simulink model "uniciclo_clot"  (R2020a)
settings: Solver=VariableStepAuto  StartTime=0.0  StopTime=Inf  MaxStep=0.01  RelTol=1e-3
InitFcn:
  | init_uniciclo
StopFcn:
  | stop_uniciclo
values from neighbouring files (symbols this model uses):
  centro = [points(1); points(2)]    [init_uniciclo.m]
  dir_retta = [cos(pi/4); sin(pi/4)]    [init_uniciclo.m]
  K1 = [40; 40]    [init_uniciclo.m]
  K2 = [50; 50]    [init_uniciclo.m]
  Lsofar = [Lsofar; sum(Lenghts)]    [init_uniciclo.m]
  Ltot = sum(Lenghts)    [init_uniciclo.m]
  n_p = length(points)    [init_uniciclo.m]
  s_finale = norm(traslazione,2)    [init_uniciclo.m]
  theta_iniziale = pi/3    (= 1.0471975512)    [init_uniciclo.m]
  theta_rette = [theta_rette ; theta_rette(n_p-2)+pi]    [init_uniciclo.m]
  v_dot_sat = 5    [init_uniciclo.m]
  v_iniziale = 1    [init_uniciclo.m]
  v_r = v_rif    (= 1)    [init_uniciclo.m]
  w_sat = 3*pi    (= 9.42477796077)    [init_uniciclo.m]
  x_p_iniziale = points(1)    [init_uniciclo.m]
  xp = points(:,1)    [init_uniciclo.m]
  y_p_iniziale = points(2)    [init_uniciclo.m]
  yp = points(:,2)    [init_uniciclo.m]
undefined symbols (not defined in the file or in its folder): indexclot, Lsofarclot
libraries: simulink x1
settings Model: Creator=Andrea_Ferroni  LastModifiedBy=Andrea_Ferroni
settings SolverCC: ZeroCrossAlgorithm=Adaptive
settings DebuggingCC: MaskedZcDiagnostic=none  IgnoredZcDiagnostic=none

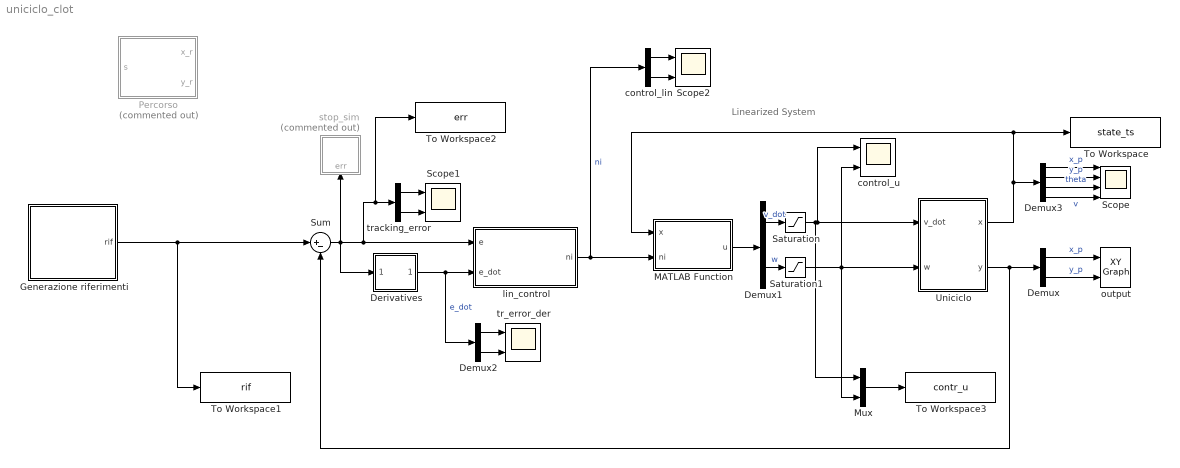
== system uniciclo_clot ==
  note: Linearized System
  Demux : Demux  Outputs=2
  Demux1 : Demux  Outputs=2
  Demux2 : Demux  Outputs=2
  Demux3 : Demux
  Derivatives : Subsystem
  Generazione riferimenti : Subsystem  Variant=on
  MATLAB Function : MATLAB Function  TreatAsAtomicUnit=on
  Mux : Mux  Inputs=2
  Percorso : MATLAB Function  Commented=on  TreatAsAtomicUnit=on
  Saturation : Saturate  UpperLimit=v_dot_sat  LowerLimit=-v_dot_sat
  Saturation1 : Saturate  UpperLimit=w_sat  LowerLimit=-w_sat
  Scope : Scope  NumInputPorts=4
  Scope1 : Scope  NumInputPorts=2
  Scope2 : Scope  NumInputPorts=2
  Sum : Sum  Inputs=|+-
  To Workspace : ToWorkspace  VariableName=state_ts  SaveFormat=Timeseries  SampleTime=-1
  To Workspace1 : ToWorkspace  VariableName=rif  SaveFormat=Timeseries  SampleTime=-1
  To Workspace2 : ToWorkspace  VariableName=err  SaveFormat=Timeseries  SampleTime=-1
  To Workspace3 : ToWorkspace  VariableName=contr_u  SaveFormat=Timeseries  SampleTime=-1
  Uniciclo : Subsystem
      mask Display: image('$imagefile'); % Use "Edit Image" on toolstrip to change.
  control_lin : Demux  Outputs=2
  control_u : Scope  NumInputPorts=2
  lin_control : MATLAB Function  TreatAsAtomicUnit=on
  output : simulink/Sinks/XY Graph  xmin=-50  xmax=50  ymin=-50  ymax=50  st=-1
  stop_sim : Subsystem  Commented=on
  tr_error_der : Scope  NumInputPorts=2
  tracking_error : Demux  Outputs=2
  wires:
  Uniciclo/1(x) -> Demux3/1, To Workspace/1, MATLAB Function/1(x)
  Generazione riferimenti/1(rif) -> Sum/1, To Workspace1/1
  Uniciclo/2(y) -> Demux/1, Sum/2
  lin_control/1(ni) -> control_lin/1, MATLAB Function/2(ni)  "ni"
  Sum/1 -> Derivatives/1(In1), lin_control/1(e), To Workspace2/1, tracking_error/1, stop_sim/1(err)
  Derivatives/1(Out1) -> Demux2/1, lin_control/2(e_dot)  "e_dot"
  Demux/1 -> output/1  "x_p"
  Demux/2 -> output/2  "y_p"
  Demux2/1 -> tr_error_der/1
  Demux2/2 -> tr_error_der/2
  tracking_error/1 -> Scope1/1
  tracking_error/2 -> Scope1/2
  Demux1/1 -> Saturation/1  "v_dot"
  Demux1/2 -> Saturation1/1  "w"
  control_lin/2 -> Scope2/2
  control_lin/1 -> Scope2/1
  Demux3/1 -> Scope/1  "x_p"
  Demux3/2 -> Scope/2  "y_p"
  Demux3/3 -> Scope/3  "theta"
  Demux3/4 -> Scope/4  "v"
  MATLAB Function/1(u) -> Demux1/1
  Saturation/1 -> Mux/1, Uniciclo/1(v_dot), control_u/1
  Saturation1/1 -> Mux/2, control_u/2, Uniciclo/2(w)
  Mux/1 -> To Workspace3/1

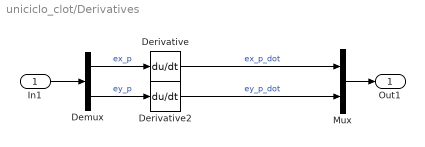
== system uniciclo_clot/Derivatives ==
  In1 : Inport
  Demux : Demux  Outputs=2
  Derivative : Derivative  CoefficientInTFapproximation=1e10
  Derivative2 : Derivative  CoefficientInTFapproximation=1e10
  Mux : Mux  Inputs=2
  Out1 : Outport
  wires:
  In1/1 -> Demux/1
  Demux/1 -> Derivative/1  "ex_p"
  Derivative/1 -> Mux/1  "ex_p_dot"
  Derivative2/1 -> Mux/2  "ey_p_dot"
  Demux/2 -> Derivative2/1  "ey_p"
  Mux/1 -> Out1/1

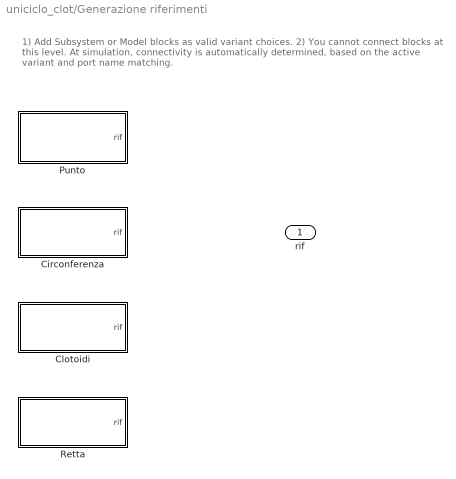
== system uniciclo_clot/Generazione riferimenti ==
  note: 1) Add Subsystem or Model blocks as valid variant choices.
      | 2) You cannot connect blocks at this level. At simulation, connectivity is automatically
      | determined, based on the active variant and port name matching.
  Circonferenza : Subsystem  VariantControl=Circonferenza
  Clotoidi : Subsystem  VariantControl=Clotoidi
  Punto : Subsystem  VariantControl=Punto
  Retta : Subsystem  VariantControl=Retta
  rif : Outport

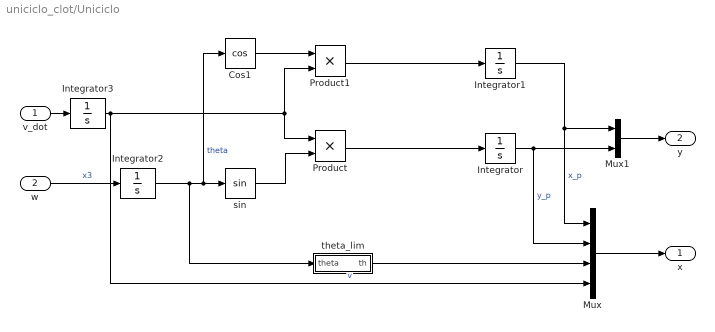
== system uniciclo_clot/Uniciclo ==
  v_dot : Inport
  w : Inport  Port=2
  Cos1 : Trigonometry  Operator=cos
  Integrator : Integrator  InitialCondition=y_p_iniziale
  Integrator1 : Integrator  InitialCondition=x_p_iniziale
  Integrator2 : Integrator  InitialCondition=theta_iniziale
  Integrator3 : Integrator  InitialCondition=v_iniziale
  Mux : Mux
  Mux1 : Mux  Inputs=2
  Product : Product
  Product1 : Product
  sin : Trigonometry
  theta_lim : MATLAB Function  TreatAsAtomicUnit=on
  x : Outport
  y : Outport  Port=2
  wires:
  v_dot/1 -> Integrator3/1
  Cos1/1 -> Product1/1
  Product1/1 -> Integrator1/1
  Product/1 -> Integrator/1
  w/1 -> Integrator2/1  "x3"
  Integrator2/1 -> theta_lim/1(theta), Cos1/1, sin/1  "theta"
  sin/1 -> Product/2
  Mux/1 -> x/1
  Integrator1/1 -> Mux/1, Mux1/1  "x_p"
  Integrator/1 -> Mux/2, Mux1/2  "y_p"
  Mux1/1 -> y/1
  Integrator3/1 -> Mux/4, Product1/2, Product/1  "v"
  theta_lim/1(th) -> Mux/3

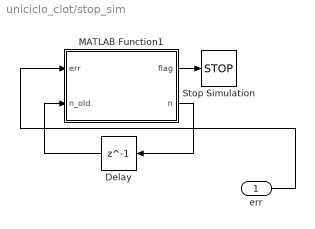
== system uniciclo_clot/stop_sim ==
  err : Inport
  Delay : Delay  DelayLength=1
  MATLAB Function1 : MATLAB Function  TreatAsAtomicUnit=on
  Stop Simulation : Stop
  wires:
  MATLAB Function1/2(n) -> Delay/1
  MATLAB Function1/1(flag) -> Stop Simulation/1
  err/1 -> MATLAB Function1/1(err)
  Delay/1 -> MATLAB Function1/2(n_old)

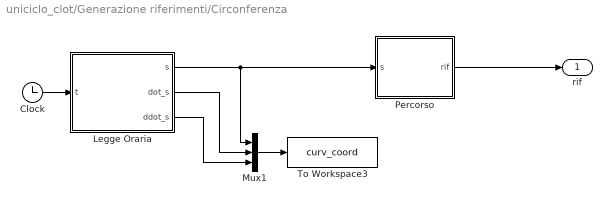
== system uniciclo_clot/Generazione riferimenti/Circonferenza ==
  Clock : Clock
  Legge Oraria : MATLAB Function  TreatAsAtomicUnit=on
  Mux1 : Mux  Inputs=3
  Percorso : MATLAB Function  TreatAsAtomicUnit=on
  To Workspace3 : ToWorkspace  VariableName=curv_coord  SaveFormat=Timeseries  SampleTime=-1
  rif : Outport
  wires:
  Legge Oraria/1(s) -> Percorso/1(s), Mux1/1
  Clock/1 -> Legge Oraria/1(t)
  Percorso/1(rif) -> rif/1
  Legge Oraria/3(ddot_s) -> Mux1/3
  Mux1/1 -> To Workspace3/1
  Legge Oraria/2(dot_s) -> Mux1/2

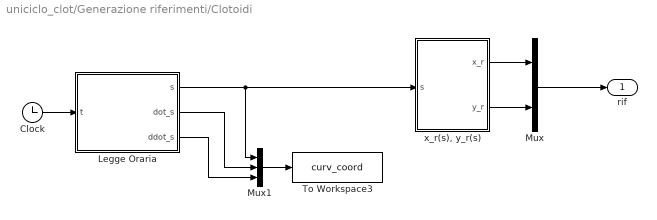
== system uniciclo_clot/Generazione riferimenti/Clotoidi ==
  Clock : Clock
  Legge Oraria : MATLAB Function  TreatAsAtomicUnit=on
  Mux : Mux  Inputs=2
  Mux1 : Mux  Inputs=3
  To Workspace3 : ToWorkspace  VariableName=curv_coord  SaveFormat=Timeseries  SampleTime=-1
  "x_r(s), y_r(s)" : MATLAB Function  TreatAsAtomicUnit=on
  rif : Outport
  wires:
  Legge Oraria/1(s) -> Mux1/1, "x_r(s), y_r(s)"/1(s)
  Legge Oraria/2(dot_s) -> Mux1/2
  Clock/1 -> Legge Oraria/1(t)
  Legge Oraria/3(ddot_s) -> Mux1/3
  Mux1/1 -> To Workspace3/1
  "x_r(s), y_r(s)"/2(y_r) -> Mux/2
  "x_r(s), y_r(s)"/1(x_r) -> Mux/1
  Mux/1 -> rif/1

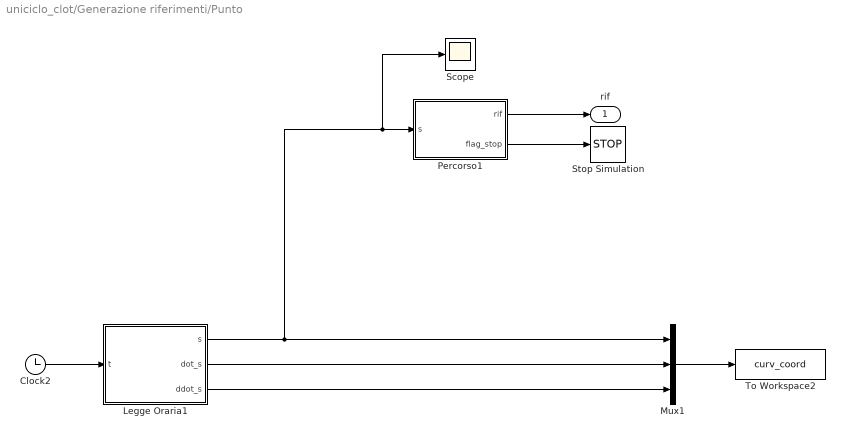
== system uniciclo_clot/Generazione riferimenti/Punto ==
  Clock2 : Clock
  Legge Oraria1 : MATLAB Function  TreatAsAtomicUnit=on
  Mux1 : Mux  Inputs=3
  Percorso1 : MATLAB Function  TreatAsAtomicUnit=on
  Scope : Scope
  Stop Simulation : Stop
  To Workspace2 : ToWorkspace  VariableName=curv_coord  SaveFormat=Timeseries  SampleTime=-1
  rif : Outport
  wires:
  Legge Oraria1/1(s) -> Mux1/1, Scope/1, Percorso1/1(s)
  Percorso1/1(rif) -> rif/1
  Percorso1/2(flag_stop) -> Stop Simulation/1
  Clock2/1 -> Legge Oraria1/1(t)
  Legge Oraria1/2(dot_s) -> Mux1/2
  Mux1/1 -> To Workspace2/1
  Legge Oraria1/3(ddot_s) -> Mux1/3

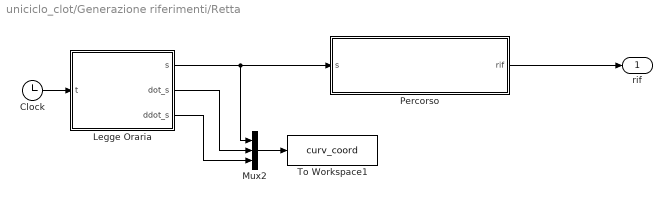
== system uniciclo_clot/Generazione riferimenti/Retta ==
  Clock : Clock
  Legge Oraria : MATLAB Function  TreatAsAtomicUnit=on
  Mux2 : Mux  Inputs=3
  Percorso : MATLAB Function  TreatAsAtomicUnit=on
  To Workspace1 : ToWorkspace  VariableName=curv_coord  SaveFormat=Timeseries  SampleTime=-1
  rif : Outport
  wires:
  Percorso/1(rif) -> rif/1
  Legge Oraria/1(s) -> Percorso/1(s), Mux2/1
  Legge Oraria/3(ddot_s) -> Mux2/3
  Mux2/1 -> To Workspace1/1
  Clock/1 -> Legge Oraria/1(t)
  Legge Oraria/2(dot_s) -> Mux2/2

== matlab function uniciclo_clot/Generazione riferimenti/Circonferenza/Percorso ==
  data: s input; rif output; centro parameter; v_r parameter
function rif = percorso(s, centro, v_r)

r = 10*v_r;  % 1
theta_circ = s/r;

if theta_circ >=  3*2*pi % dopotre giri ti fermi
	theta_circ = 3*2*pi;
end

rif = centro + r*[cos(theta_circ);sin(theta_circ)];		% circonferenza

end

== matlab function uniciclo_clot/Generazione riferimenti/Retta/Legge Oraria ==
  data: t input; s output; v_rif parameter; dot_s output; ddot_s output
function [s, dot_s, ddot_s]  = legge_oraria(t, v_rif)
%#codegen PEPO

s = v_rif*t;
dot_s = v_rif;
ddot_s = 0.0;


end

== matlab function uniciclo_clot/Generazione riferimenti/Retta/Percorso ==
  data: s input; rif output; dir_retta parameter
function rif  = retta(s, dir_retta)

rif = [0;0] + s * dir_retta;


end

== matlab function uniciclo_clot/Generazione riferimenti/Clotoidi/x_r(s), y_r(s) ==
  data: s input; x_r output size=1; y_r output size=1; indexclot parameter; theta_rette parameter; yp parameter; xp parameter; Lsofar parameter; n_p parameter; Lsofarclot parameter; Ltot parameter
function [x_r,y_r] = percorso(s, indexclot, theta_rette, yp, xp, ...
										Lsofar, n_p, Lsofarclot, Ltot)
									
coder.extrinsic('pointsOnClothoid')
% fine percorso
if s >= Ltot
	s = Ltot; % cosi` da plottare l'ultimo punto
end

ntratto=0;
	XYS = [0; 0]; %definito prima

	%Parte per capire in che tratto sono
	if s < Lsofar(1)
		ntratto=1;
	else
		for ii=2:(n_p-1)
			if s>=Lsofar(ii-1) && s<=Lsofar(ii)
				ntratto=ii;
			end
		end
	end	

		%calcolo delle coordinate x e y riferite a s e a ntratto
	if mod(ntratto,2)==1            %tratti dispari - rette
		if ntratto==1
			XYS=[xp(ntratto)+cos(theta_rette(ntratto))*(s); ...
				yp(ntratto)+sin(theta_rette(ntratto))*(s)];
		else
			srel=s-Lsofar(ntratto-1);
			XYS=[	xp(ntratto)	+ cos(theta_rette(ntratto))	* srel; ...
					yp(ntratto)	+ sin(theta_rette(ntratto))	* srel];
		end 

	elseif mod(ntratto,2)==0	%tratti pari - clotoidi
		srel=s-Lsofar(ntratto-1);

		if srel<=Lsofarclot(ntratto/2).Lclot(1)
			XYS = double(pointsOnClothoid( indexclot(ntratto/2).clot.S0, srel ));

		elseif srel>Lsofarclot(ntratto/2).Lclot(1) & srel<=Lsofarclot(ntratto/2).Lclot(2)
			XYS = double(pointsOnClothoid( indexclot(ntratto/2).clot.SM, srel- indexclot(ntratto/2).clot.S0.L ));

		elseif srel>Lsofarclot(ntratto/2).Lclot(2)
			XYS = double(pointsOnClothoid( indexclot(ntratto/2).clot.S1, srel- indexclot(ntratto/2).clot.S0.L - indexclot(ntratto/2).clot.SM.L ));
		end

		%XYS = double(pointsOnClothoid( indexclot(ntratto/2).clot, s-Lsofar(ntratto-1) ));
	end

	x_r = XYS(1);
	y_r = XYS(2);
%--------------------------------------------------
% end function
end

== matlab function uniciclo_clot/Generazione riferimenti/Punto/Legge Oraria1 ==
  data: t input; s output; v_rif parameter; dot_s output; ddot_s output
function [s, dot_s, ddot_s]  = legge_oraria(t, v_rif)
%#codegen PEPO

s = v_rif*t;
dot_s = v_rif;
ddot_s = 0.0;


end

== matlab function uniciclo_clot/Generazione riferimenti/Punto/Percorso1 ==
  data: s input; rif output; dir_retta parameter; x_p_iniziale parameter; y_p_iniziale parameter; s_finale parameter; flag_stop output
function [rif, flag_stop] = retta(s, dir_retta, x_p_iniziale, y_p_iniziale, s_finale)

if s >= s_finale
	s = s_finale;
	flag_stop = 1;
else
	flag_stop = 0;
end

rif = [x_p_iniziale; y_p_iniziale] + s * dir_retta;




end

== matlab function uniciclo_clot/lin_control ==
  data: e input; ni output; e_dot input; K1 parameter size=[2,1]; K2 parameter size=[2,1]
function ni = lin_control(e, e_dot, K1, K2)

ni = K1.*e + K2.*e_dot;

end

== matlab function uniciclo_clot/MATLAB Function ==
  data: x input; ni input; u output
function u = Linearized(x,ni)
theta = x(3);
v = x(4);

E_inv = inv_E(theta, v);
G = Gamma();
u =  -E_inv*G + E_inv*ni;
end

% gamma
function Gm = Gamma()
Gm = [0;0];
end
% 
function E_in = inv_E(theta, v)
E = [cos(theta) -v*sin(theta);
	 sin(theta)  v*cos(theta)];
E_in = inv(E);
end

== matlab function uniciclo_clot/Uniciclo/theta_lim ==
  data: theta input; th output
function th = theta_lim(theta)
c = cos(theta);
s = sin(theta);
th = atan2(s, c);

== matlab function uniciclo_clot/stop_sim/MATLAB Function1 ==
  data: flag output; err input; n output; n_old input; threshold parameter
function [flag, n] = stop_function(err, n_old, threshold)
	flag = 0;
	n = n_old;
	if norm(err, 2) < threshold
		n=n+1;
	else
		n=0;
	end
	
	if n > 500
		flag = 1;
		n = 0;
	end
end

== matlab function uniciclo_clot/Generazione riferimenti/Clotoidi/Legge Oraria ==
  data: t input; s output; v_rif parameter; dot_s output; ddot_s output
function [s, dot_s, ddot_s]  = legge_oraria(t, v_rif)
%#codegen PEPO

s = v_rif*t;
dot_s = v_rif;
ddot_s = 0.0;


end

== matlab function uniciclo_clot/Percorso ==
  data: s input; x_r output; y_r output
function [x_r, y_r] = percorso(s)



% pos = s * [0; 1] + [1; 0]*cos(s);				% sinusoide

r = 10;
theta_circ = s/r;

pos = r*[cos(theta_circ);sin(theta_circ)];		% circonferenza
%p = [cos(s/2);sin(s/2)];
%pos = min(1/(s/100+0.01),r) * p;					% spirale
%pos = 1/(s/100+0.01) * p;

x_r = pos(1);
y_r = pos(2);

end

== matlab function uniciclo_clot/Generazione riferimenti/Circonferenza/Legge Oraria ==
  data: t input; s output; v_rif parameter; dot_s output; ddot_s output
function [s, dot_s, ddot_s]  = legge_oraria(t, v_rif)
%#codegen PEPO

s = v_rif*t;
dot_s = v_rif;
ddot_s = 0.0;


end
